simulink model "lab_otu_observer2022"  (R2023a)
settings: Solver=VariableStepAuto  StartTime=0.0  StopTime=10.0  RelTol=1e-3
undefined symbols (not defined in the file): A, B, C, D
libraries: simulink x2
settings Model: Creator=Student  LastModifiedBy=gnomy
settings SolverCC: AlgebraicLoopSolver=TrustRegion
settings RTWCC: DLArmComputeVersion=19.05

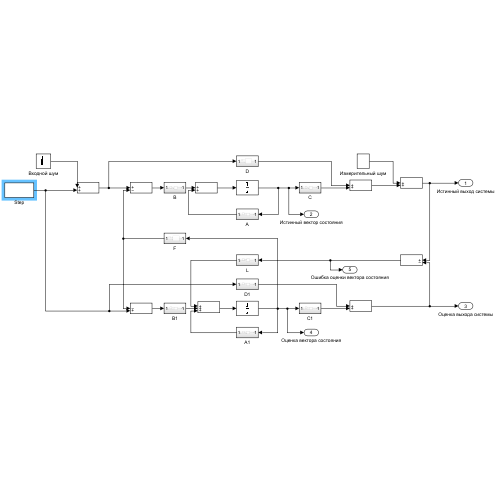
[thumbnail: Simulink's stored preview of the top-level diagram]
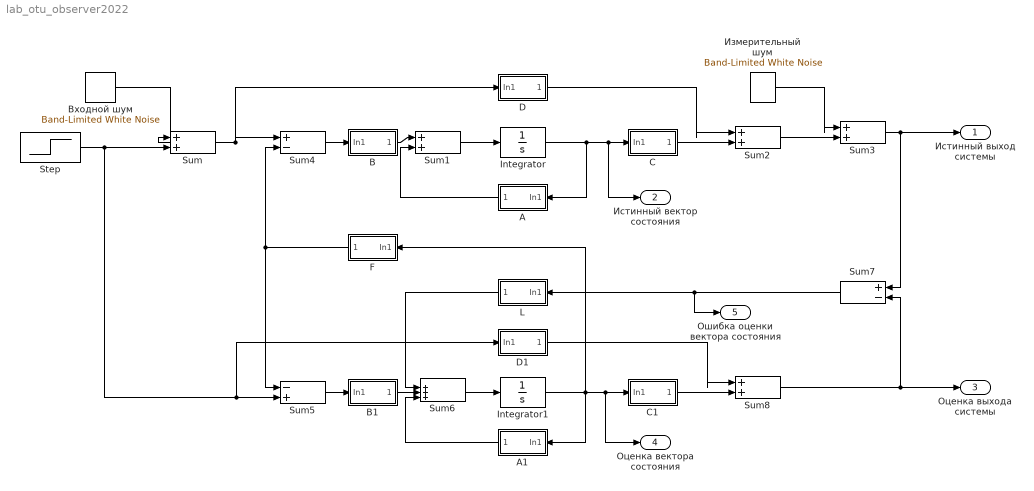
== system lab_otu_observer2022 ==
  A : Subsystem
      settings: PortSchema="{\"entries\":[{\"content\":{\"sides\":[{\"content\":{\"connectorIds\":[\"Out1\"]},\"type\":\"ConnectorPlacement.EquallySpacedRectSide\",\"uuid\":\"553fa999-2026-4954-8d58-e45988c3f902\"},{\"content\":{\"connectorIds\":[\"In1\"],\"side\":\"RIGHT\"},\"type\":\"ConnectorPlacement.EquallySpacedRectSide\",\"uuid\":\"47cbfa4f-fe07-47a2-a7c5-8d72da3022ae\"},{\"content\":{\"side\":\"TOP\"},\"type\":\"ConnectorPlacement.EquallySpacedRectSide\",\"uuid\":\"1fb97f4a-5d60-499d-8ca4-1578e218951b\"}]},\"type\":\"ConnectorPlacement.EquallySpacedConnector\",\"uuid\":\"74d96124-15bd-4fa6-8e02-0bf4e721d4df\"}],\"packageUris\":[\"http://schema.mathworks.com/mf0/Connector/R2020b\"],\"version\":\"1.0\"}"
  A1 : Subsystem
      settings: PortSchema="{\"entries\":[{\"content\":{\"sides\":[{\"content\":{\"connectorIds\":[\"Out1\"]},\"type\":\"ConnectorPlacement.EquallySpacedRectSide\",\"uuid\":\"553fa999-2026-4954-8d58-e45988c3f902\"},{\"content\":{\"connectorIds\":[\"In1\"],\"side\":\"RIGHT\"},\"type\":\"ConnectorPlacement.EquallySpacedRectSide\",\"uuid\":\"47cbfa4f-fe07-47a2-a7c5-8d72da3022ae\"},{\"content\":{\"side\":\"TOP\"},\"type\":\"ConnectorPlacement.EquallySpacedRectSide\",\"uuid\":\"1fb97f4a-5d60-499d-8ca4-1578e218951b\"}]},\"type\":\"ConnectorPlacement.EquallySpacedConnector\",\"uuid\":\"74d96124-15bd-4fa6-8e02-0bf4e721d4df\"}],\"packageUris\":[\"http://schema.mathworks.com/mf0/Connector/R2020b\"],\"version\":\"1.0\"}"
  B : Subsystem
  B1 : Subsystem
  C : Subsystem
  C1 : Subsystem
  D : Subsystem
  D1 : Subsystem
  F : Subsystem
      settings: PortSchema="{\"entries\":[{\"content\":{\"sides\":[{\"content\":{\"connectorIds\":[\"Out1\"]},\"type\":\"ConnectorPlacement.EquallySpacedRectSide\",\"uuid\":\"553fa999-2026-4954-8d58-e45988c3f902\"},{\"content\":{\"connectorIds\":[\"In1\"],\"side\":\"RIGHT\"},\"type\":\"ConnectorPlacement.EquallySpacedRectSide\",\"uuid\":\"47cbfa4f-fe07-47a2-a7c5-8d72da3022ae\"},{\"content\":{\"side\":\"TOP\"},\"type\":\"ConnectorPlacement.EquallySpacedRectSide\",\"uuid\":\"1fb97f4a-5d60-499d-8ca4-1578e218951b\"}]},\"type\":\"ConnectorPlacement.EquallySpacedConnector\",\"uuid\":\"74d96124-15bd-4fa6-8e02-0bf4e721d4df\"}],\"packageUris\":[\"http://schema.mathworks.com/mf0/Connector/R2020b\"],\"version\":\"1.0\"}"
  Integrator : Integrator
  Integrator1 : Integrator
  L : Subsystem
      settings: PortSchema="{\"entries\":[{\"content\":{\"sides\":[{\"content\":{\"connectorIds\":[\"Out1\"]},\"type\":\"ConnectorPlacement.EquallySpacedRectSide\",\"uuid\":\"553fa999-2026-4954-8d58-e45988c3f902\"},{\"content\":{\"connectorIds\":[\"In1\"],\"side\":\"RIGHT\"},\"type\":\"ConnectorPlacement.EquallySpacedRectSide\",\"uuid\":\"47cbfa4f-fe07-47a2-a7c5-8d72da3022ae\"},{\"content\":{\"side\":\"TOP\"},\"type\":\"ConnectorPlacement.EquallySpacedRectSide\",\"uuid\":\"1fb97f4a-5d60-499d-8ca4-1578e218951b\"}]},\"type\":\"ConnectorPlacement.EquallySpacedConnector\",\"uuid\":\"74d96124-15bd-4fa6-8e02-0bf4e721d4df\"}],\"packageUris\":[\"http://schema.mathworks.com/mf0/Connector/R2020b\"],\"version\":\"1.0\"}"
  Step : Step  SampleTime=0.01  VectorParams1D=off
  Sum{,1..3,8} (5 alike) : Sum  Inputs=|++
  Sum4 : Sum  Inputs=|+-
  Sum5 : Sum  Inputs=|-+
  Sum6 : Sum  Inputs=|+++
  Sum7 : Sum  Inputs=|+-
  Входной шум : simulink/Sources/Band-Limited White Noise  Cov=1e-06  Ts=0.01  seed=[23341]
  Измерительный шум : simulink/Sources/Band-Limited White Noise  Cov=1e-05  Ts=0.01  seed=[23341]
  Истинный выход системы : Outport
  Истинный вектор состояния : Outport  Port=2
  Оценка выхода системы : Outport  Port=3
  Оценка вектора состояния : Outport  Port=4
  Ошибка оценки вектора состояния : Outport  Port=5
  wires:
  Входной шум/1 -> Sum/1
  Step/1 -> D1/1(In1), Sum5/2, Sum/2
  Sum1/1 -> Integrator/1
  A/1(Out1) -> Sum1/2
  Integrator/1 -> A/1(In1), Истинный вектор состояния/1, C/1(In1)
  C/1(Out1) -> Sum2/2
  Sum2/1 -> Sum3/2
  Измерительный шум/1 -> Sum3/1
  Sum/1 -> D/1(In1), Sum4/1
  Sum4/1 -> B/1(In1)
  B/1(Out1) -> Sum1/1
  F/1(Out1) -> Sum5/1, Sum4/2
  Sum5/1 -> B1/1(In1)
  B1/1(Out1) -> Sum6/2
  Sum6/1 -> Integrator1/1
  L/1(Out1) -> Sum6/1
  Integrator1/1 -> A1/1(In1), F/1(In1), Оценка вектора состояния/1, C1/1(In1)
  Sum7/1 -> Ошибка оценки вектора состояния/1, L/1(In1)
  Sum3/1 -> Истинный выход системы/1, Sum7/1
  C1/1(Out1) -> Sum8/2
  D1/1(Out1) -> Sum8/1
  Sum8/1 -> Оценка выхода системы/1, Sum7/2
  A1/1(Out1) -> Sum6/3
  D/1(Out1) -> Sum2/1

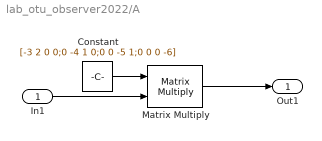
== system lab_otu_observer2022/A ==
  In1 : Inport
  Constant : Constant  Value=[-3 2 0 0;0 -4 1 0;0 0 -5 1;0 0 0 -6]  VectorParams1D=off
  Matrix Multiply : Product  Multiplication=Matrix(*)
  Out1 : Outport
  wires:
  In1/1 -> Matrix Multiply/2
  Matrix Multiply/1 -> Out1/1
  Constant/1 -> Matrix Multiply/1

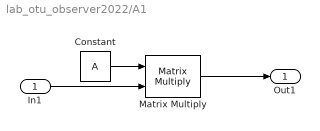
== system lab_otu_observer2022/A1 ==
  In1 : Inport
  Constant : Constant  Value=A  VectorParams1D=off
  Matrix Multiply : Product  Multiplication=Matrix(*)
  Out1 : Outport
  wires:
  In1/1 -> Matrix Multiply/2
  Matrix Multiply/1 -> Out1/1
  Constant/1 -> Matrix Multiply/1

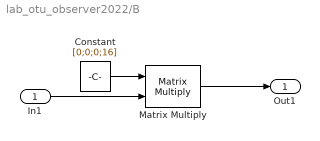
== system lab_otu_observer2022/B ==
  In1 : Inport
  Constant : Constant  Value=[0;0;0;16]  VectorParams1D=off
  Matrix Multiply : Product  Multiplication=Matrix(*)
  Out1 : Outport
  wires:
  In1/1 -> Matrix Multiply/2
  Matrix Multiply/1 -> Out1/1
  Constant/1 -> Matrix Multiply/1

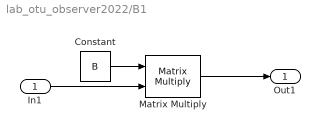
== system lab_otu_observer2022/B1 ==
  In1 : Inport
  Constant : Constant  Value=B  VectorParams1D=off
  Matrix Multiply : Product  Multiplication=Matrix(*)
  Out1 : Outport
  wires:
  In1/1 -> Matrix Multiply/2
  Matrix Multiply/1 -> Out1/1
  Constant/1 -> Matrix Multiply/1

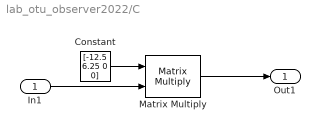
== system lab_otu_observer2022/C ==
  In1 : Inport
  Constant : Constant  Value=[-12.5 6.25 0 0]  VectorParams1D=off
  Matrix Multiply : Product  Multiplication=Matrix(*)
  Out1 : Outport
  wires:
  In1/1 -> Matrix Multiply/2
  Matrix Multiply/1 -> Out1/1
  Constant/1 -> Matrix Multiply/1

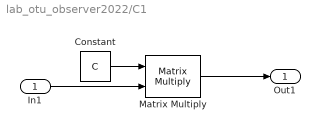
== system lab_otu_observer2022/C1 ==
  In1 : Inport
  Constant : Constant  Value=C  VectorParams1D=off
  Matrix Multiply : Product  Multiplication=Matrix(*)
  Out1 : Outport
  wires:
  In1/1 -> Matrix Multiply/2
  Matrix Multiply/1 -> Out1/1
  Constant/1 -> Matrix Multiply/1

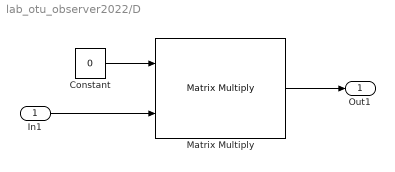
== system lab_otu_observer2022/D ==
  In1 : Inport
  Constant : Constant  Value=0  VectorParams1D=off
  Matrix Multiply : Product  Multiplication=Matrix(*)
  Out1 : Outport
  wires:
  Constant/1 -> Matrix Multiply/1
  Matrix Multiply/1 -> Out1/1
  In1/1 -> Matrix Multiply/2

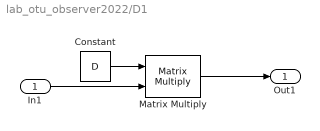
== system lab_otu_observer2022/D1 ==
  In1 : Inport
  Constant : Constant  Value=D  VectorParams1D=off
  Matrix Multiply : Product  Multiplication=Matrix(*)
  Out1 : Outport
  wires:
  In1/1 -> Matrix Multiply/2
  Matrix Multiply/1 -> Out1/1
  Constant/1 -> Matrix Multiply/1

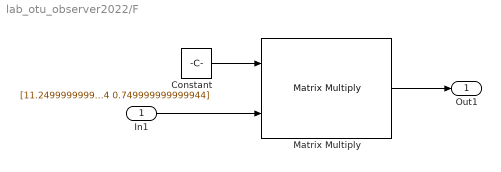
== system lab_otu_observer2022/F ==
  In1 : Inport
  Constant : Constant  Value=[11.2499999999979 14.9999999999976 4.49999999999944 0.749999999999944]  VectorParams1D=off
  Matrix Multiply : Product  Multiplication=Matrix(*)
  Out1 : Outport
  wires:
  In1/1 -> Matrix Multiply/2
  Matrix Multiply/1 -> Out1/1
  Constant/1 -> Matrix Multiply/1

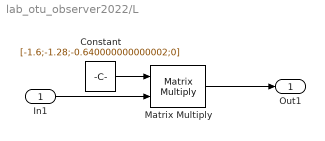
== system lab_otu_observer2022/L ==
  In1 : Inport
  Constant : Constant  Value=[-1.6;-1.28;-0.640000000000002;0]  VectorParams1D=off
  Matrix Multiply : Product  Multiplication=Matrix(*)
  Out1 : Outport
  wires:
  In1/1 -> Matrix Multiply/2
  Matrix Multiply/1 -> Out1/1
  Constant/1 -> Matrix Multiply/1
